simulink model "Commander_Stabilizer_Qdrone_serial"  (R2019a)
settings: Solver=ode2  StartTime=0.0  StopTime=inf  FixedStep=0.001  RelTol=1e-3  EnableMultiTasking=on
InitFcn:
  | set_param(gcs, 'ZoomFactor','FitSystem')
model workspace (MAT data in the model file):
  target_system = 1
undefined symbols (not defined in the file or in its folder): HIL, qc_get_step_size
libraries: quarc_library x53, simulink x24, simulink_extras x4
(part 2 of 4)

== system Commander_Stabilizer_Qdrone_serial/HORIZON FRAME CONVERSION AND ESTIMATION/Estimate Yaw Angle ==
  note: Improve Yaw Estimate
  note: The complementary filters for yaw estimation uses an accurate but noisy yaw approximation to correct the drifting integral of the fast gyroscopic rate to yield an accurate and fast yaw estimate.
  Yaw Rate (rad/s) : Inport
  Yaw Correction (rad) : Inport  Port=2
  Reset : Inport  Port=3
  Integrator1 : Integrator
  Integrator2 : Integrator  ExternalReset=rising
  Ki1 : Gain  Gain=0.1
  Kp1 : Gain
  Sum1 : Sum  Inputs=|-+
  Sum2 : Sum  Inputs=+--
  Yaw Estimate (rad) : Outport
  wires:
  Yaw Rate (rad/s)/1 -> Sum2/1
  Sum1/1 -> Ki1/1, Kp1/1
  Kp1/1 -> Sum2/2
  Reset/1 -> Integrator2/2
  Sum2/1 -> Integrator1/1
  Ki1/1 -> Integrator2/1
  Integrator1/1 -> Yaw Estimate (rad)/1, Sum1/2
  Integrator2/1 -> Sum2/3
  Yaw Correction (rad)/1 -> Sum1/1

== system Commander_Stabilizer_Qdrone_serial/HORIZON FRAME CONVERSION AND ESTIMATION/Pose Rate Estimation ==
  note: Second order filter + Derivative
  note: Generate Pose Rate Approximation
  note: Improve Position Rate Estimate
  note: Complementary Filter implementation (similar to those in the Stabilizer module)
  note: The complementary filter uses an accurate but noisy pose rate approximation to correct the drifting integral of the fast accelerometer readings to yield an accurate and fast pose rate estimate.
  HF Vehicle Acceleration (m/s/s) [3] : Inport
  "HF Pose Measurement (m, rad) [4]" : Inport  Port=2
  Yaw Rate (rad/s) : Inport  Port=3
  Reset : Inport  Port=4
  Integrator6 : Integrator
  Integrator7 : Integrator  ExternalReset=rising
  Ki3 : Gain  Gain=0.1
  Kp3 : Gain
  Mux2 : Mux  Inputs=2
  Second-Order Low-Pass Filter : quarc_library/Continuous/Second-Order Low-Pass Filter  params_source=External (input ports)  input_width=1  input_zeta=1  input_init=0
  Selector : Selector  InputPortWidth=4  IndexOptions=Index vector (dialog)  Indices=[1:3]  OutputSizes=1
  Sum8 : Sum  Inputs=|-+
  Sum9 : Sum  Inputs=+--
  Terminator1 : Terminator
  wn : Constant  Value=50
  zt : Constant
  "HF Pose Rate Estimate (m/s, rad/s) [4]" : Outport
  wires:
  "HF Pose Measurement (m, rad) [4]"/1 -> Selector/1
  Yaw Rate (rad/s)/1 -> Mux2/2
  Reset/1 -> Integrator7/2
  Integrator7/1 -> Sum9/3
  Integrator6/1 -> Sum8/2, Mux2/1
  Kp3/1 -> Sum9/2
  Ki3/1 -> Integrator7/1
  Sum8/1 -> Kp3/1, Ki3/1
  Sum9/1 -> Integrator6/1
  Mux2/1 -> "HF Pose Rate Estimate (m/s, rad/s) [4]"/1
  wn/1 -> Second-Order Low-Pass Filter/2
  Second-Order Low-Pass Filter/1 -> Terminator1/1
  Second-Order Low-Pass Filter/2 -> Sum8/1
  zt/1 -> Second-Order Low-Pass Filter/3
  HF Vehicle Acceleration (m/s/s) [3]/1 -> Sum9/1
  Selector/1 -> Second-Order Low-Pass Filter/4, Second-Order Low-Pass Filter/1

== system Commander_Stabilizer_Qdrone_serial/HORIZON FRAME CONVERSION AND ESTIMATION/Transform from Body Frame to Horizon Frame ==
  note: Accelerometer Reading + Gravity = Vehicle Acceleration
  HF_R_BF : Inport
  BF Net Acceleration (m/s/s) [3] : Inport  Port=2
  Product : Product  Multiplication=Matrix(*)
  gravity correction : Bias  Bias=[0 0 -9.81]
  HF Vehicle Acceleration (m/s/s) [3] : Outport
  wires:
  gravity correction/1 -> HF Vehicle Acceleration (m/s/s) [3]/1  "HF Vehicle Acceleration"
  HF_R_BF/1 -> Product/1
  BF Net Acceleration (m/s/s) [3]/1 -> Product/2
  Product/1 -> gravity correction/1  "HF Accelerometer Reading"

== system Commander_Stabilizer_Qdrone_serial/HORIZON FRAME CONVERSION AND ESTIMATION/Transform from Inertial Frame to Horizon Frame ==
  HF_R_IF : Inport
  "IF Pose Command (m, rad) [4]" : Inport  Port=2
  Yaw Estimate : Inport  Port=3
  "IF Pose Measurement (m, rad) [4]" : Inport  Port=4
  Mux1 : Mux  Inputs=2
  Mux3 : Mux  Inputs=2
  Product1 : Product  Multiplication=Matrix(*)
  Product2 : Product  Multiplication=Matrix(*)
  Select Position Command : Selector  InputPortWidth=4  IndexOptions=Index vector (dialog)  Indices=1:3  OutputSizes=1
  Select Position Estimate : Selector  InputPortWidth=4  IndexOptions=Index vector (dialog)  Indices=1:3  OutputSizes=1
  Select Yaw Command : Selector  InputPortWidth=4  IndexOptions=Index vector (dialog)  Indices=4  OutputSizes=1
  "HF Pose Estimate (m, rad) [4]" : Outport
  "HF Pose Command (m, rad) [4]" : Outport  Port=2
  wires:
  Yaw Estimate/1 -> Mux1/2
  "IF Pose Command (m, rad) [4]"/1 -> Select Position Command/1, Select Yaw Command/1
  Select Position Command/1 -> Product1/2  "IF Position Command"
  Product2/1 -> Mux1/1  "HF Position Measurement"
  Product1/1 -> Mux3/1  "HF Position Command"
  Mux3/1 -> "HF Pose Command (m, rad) [4]"/1
  Mux1/1 -> "HF Pose Estimate (m, rad) [4]"/1
  HF_R_IF/1 -> Product2/1, Product1/1
  Select Yaw Command/1 -> Mux3/2
  Select Position Estimate/1 -> Product2/2  "IF Position Measurement"
  "IF Pose Measurement (m, rad) [4]"/1 -> Select Position Estimate/1

== system Commander_Stabilizer_Qdrone_serial/STABILIZER - QDRONE /BLACKBOX ==
  Mode : Inport
  Controller Log : Inport  Port=2
  Plant Log : Inport  Port=3
  Safety Log : Inport  Port=4
  Mux : Mux
  To Host File : quarc_library/Sinks/To Host/To Host File  file_name=saved_data/%m/Stabilizer_%{date}_%{time}.mat  variable_name=stabilizer_data  decimation=1  sample_time=-1  file_format=MAT-file v.5  options=No header or footer  append=off  final_file_name=saved_data/Commander_Stabilizer_Qdrone_serial/Stabilizer_04-Apr-2021_22-18-28.mat  bitrate=2000000
      settings: SourceProductName=The database C:\Users\user\AppData\Roaming\MathWorks\MATLAB\R2017a\slblocks_master.db is locked, or a table in the database is locked. (database is locked)
  wires:
  Mux/1 -> To Host File/1
  Safety Log/1 -> Mux/1
  Controller Log/1 -> Mux/2
  Plant Log/1 -> Mux/3
  Mode/1 -> Mux/4

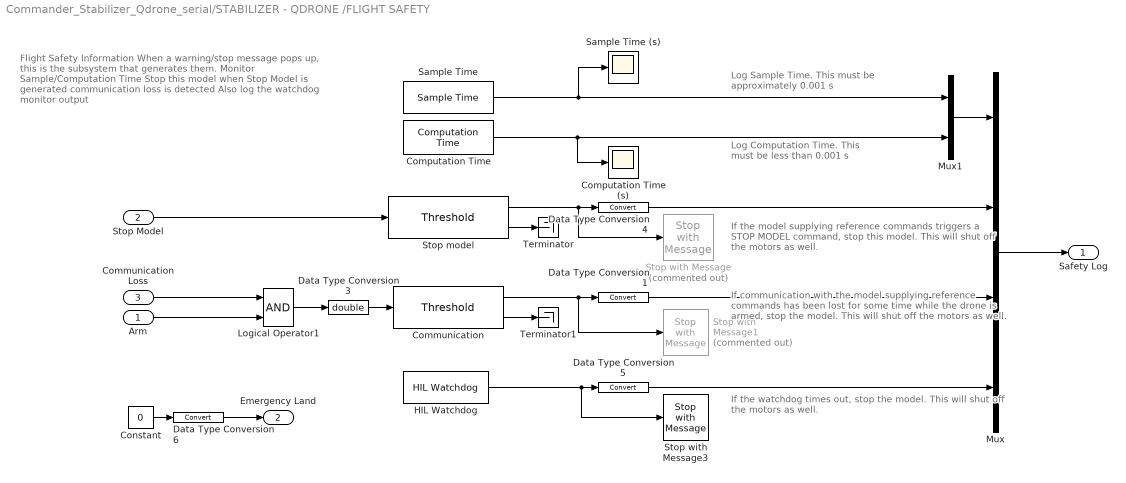
== system Commander_Stabilizer_Qdrone_serial/STABILIZER - QDRONE /FLIGHT SAFETY ==
  note: Flight Safety Information
      |
      | When a warning/stop message pops up, this is the subsystem
      | that generates them.
      |
      | Monitor Sample/Computation Time
      | Stop this model
      | when Stop Model is generated
      | communication loss is detected
      | Also log the watchdog monitor output
  note: Log Sample Time. This must be approximately 0.001 s
  note: Log Computation Time. This must be less than 0.001 s
  note: If the model supplying reference commands triggers a STOP MODEL command, stop this model. This will shut off the motors as well.
  note: If communication with the model supplying reference commands has been lost for some time while the drone is armed, stop the model. This will shut off the motors as well.
  note: If the watchdog times out, stop the model. This will shut off the motors as well.
  Arm : Inport
  Stop Model : Inport  Port=2
  Communication Loss : Inport  Port=3
  Communication : quarc_library/Discontinuities/Threshold  operator=>=  param_src=Specify via dialog  threshold=0.5  duration=1
      settings: SourceProductName=The database C:\Users\user\AppData\Roaming\MathWorks\MATLAB\R2017a\slblocks_master.db is locked, or a table in the database is locked. (database is locked)
  Computation Time : quarc_library/Sources/Time/Computation Time  sample_time=qc_get_step_size  use_model=on  use_cpu_time=off
      settings: SourceProductName=The database C:\Users\user\AppData\Roaming\MathWorks\MATLAB\R2017a\slblocks_master.db is locked, or a table in the database is locked. (database is locked)
  Computation Time (s) : Scope
  Constant : Constant  Value=0
  Data Type Conversion{1,4..6} (4 alike) : DataTypeConversion
  Data Type Conversion3 : DataTypeConversion  OutDataTypeStr=double
  HIL Watchdog : quarc_library/Data Acquisition/Generic/Watchdog/HIL Watchdog  object_name=HIL-1  timeout=0.1  sample_time=qc_get_step_size  active=off
      settings: AttributesFormatString=(%<object_name>)  SourceProductName=QUARC Targets
  Logical Operator1 : Logic  AllPortsSameDT=off  OutDataTypeStr=boolean
  Mux : Mux
  Mux1 : Mux  Inputs=2
  Sample Time : quarc_library/Sources/Time/Sample Time  Priority=-99  sample_time=qc_get_step_size
      settings: SourceProductName=The database C:\Users\user\AppData\Roaming\MathWorks\MATLAB\R2017a\slblocks_master.db is locked, or a table in the database is locked. (database is locked)
  Sample Time (s) : Scope
  Stop model : quarc_library/Discontinuities/Threshold  operator=>=  param_src=Specify via dialog  threshold=0.5  duration=0.1
      settings: SourceProductName=The database C:\Users\user\AppData\Roaming\MathWorks\MATLAB\R2017a\slblocks_master.db is locked, or a table in the database is locked. (database is locked)
  Stop with Message : quarc_library/Sinks/Error Handling/Stop with Message  Commented=on  message_type=Fixed error message  message_icon=Information  message=QDrone Stabilizer: Commander Terminated
      settings: SourceProductName=The database C:\Users\user\AppData\Roaming\MathWorks\MATLAB\R2017a\slblocks_master.db is locked, or a table in the database is locked. (database is locked)
  Stop with Message1 : quarc_library/Sinks/Error Handling/Stop with Message  Commented=on  message_type=Fixed error message  message_icon=Warning  message=QDrone Stabilizer: Communication with Commander lost
      settings: SourceProductName=The database C:\Users\user\AppData\Roaming\MathWorks\MATLAB\R2017a\slblocks_master.db is locked, or a table in the database is locked. (database is locked)
  Stop with Message3 : quarc_library/Sinks/Error Handling/Stop with Message  message_type=Fixed error message  message_icon=Information  message=QDrone Stabilizer: HIL Watchdog timer expired
      settings: SourceProductName=The database C:\Users\user\AppData\Roaming\MathWorks\MATLAB\R2017a\slblocks_master.db is locked, or a table in the database is locked. (database is locked)
  Terminator : Terminator
  Terminator1 : Terminator
  Safety Log : Outport
  Emergency Land : Outport  Port=2
  wires:
  Mux/1 -> Safety Log/1
  Computation Time/1 -> Computation Time (s)/1, Mux1/2
  Sample Time/1 -> Sample Time (s)/1, Mux1/1
  Data Type Conversion4/1 -> Mux/2
  HIL Watchdog/1 -> Stop with Message3/1, Data Type Conversion5/1
  Stop model/2 -> Terminator/1
  Stop model/1 -> Data Type Conversion4/1, Stop with Message/1
  Stop Model/1 -> Stop model/1
  Communication/2 -> Terminator1/1
  Logical Operator1/1 -> Data Type Conversion3/1
  Data Type Conversion1/1 -> Mux/3
  Arm/1 -> Logical Operator1/2
  Communication/1 -> Data Type Conversion1/1, Stop with Message1/1
  Data Type Conversion3/1 -> Communication/1
  Communication Loss/1 -> Logical Operator1/1
  Mux1/1 -> Mux/1
  Constant/1 -> Data Type Conversion6/1
  Data Type Conversion6/1 -> Emergency Land/1
  Data Type Conversion5/1 -> Mux/4

== system Commander_Stabilizer_Qdrone_serial/STABILIZER - QDRONE /MODE SWITCHBOX ==
  note: This subsystem switches between Attitude Torques AND Attitude Commands depending on
      | the value of the Mode signal:
      | Mode = 1	=> 		Torque mode, Attitude Commands are zeroed
      | Mode = 0	=> 		Angle mode, Attitude Torques are zeroed
  Mode (0,1) : Inport
  Attitude Torques : Inport  Port=2
  Attitude Commands : Inport  Port=3
  Switch : Switch  Criteria=u2 > Threshold  Threshold=0.5
  Switch1 : Switch  Criteria=u2 > Threshold  Threshold=0.5
  Zero Torque/Command : Constant  Value=[0 0 0]
  Attitude Torques (Nm) [3] : Outport
  "Attitude Commands (rad, rad/s) [3]" : Outport  Port=2
  wires:
  Zero Torque/Command/1 -> Switch1/1, Switch/3
  Attitude Torques/1 -> Switch/1
  Switch/1 -> Attitude Torques (Nm) [3]/1
  Mode (0,1)/1 -> Switch1/2, Switch/2
  Switch1/1 -> "Attitude Commands (rad, rad/s) [3]"/1
  Attitude Commands/1 -> Switch1/3

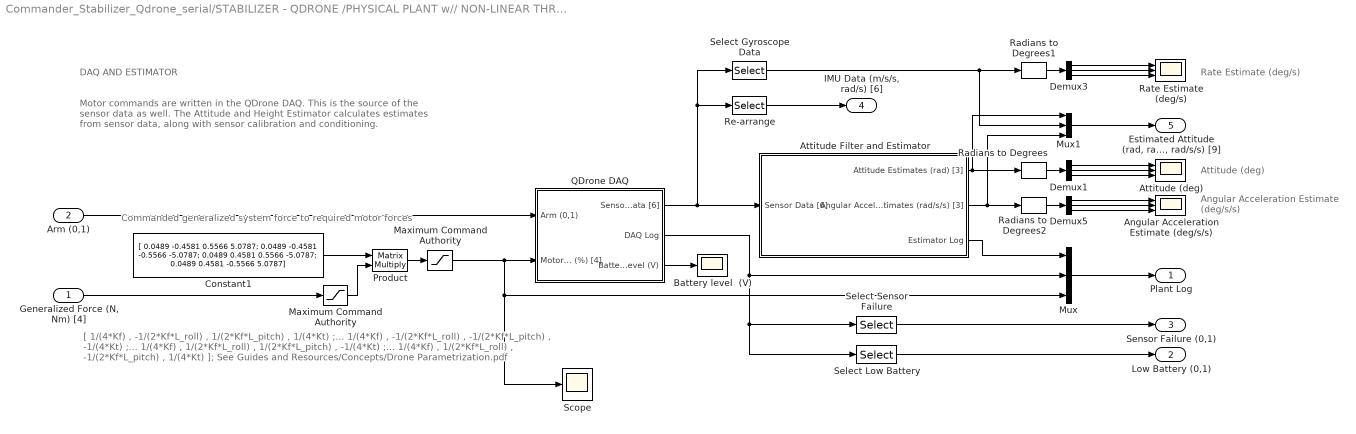
== system Commander_Stabilizer_Qdrone_serial/STABILIZER - QDRONE /PHYSICAL PLANT w// NON-LINEAR THRUST ==
  note: [ 1/(4*Kf) , -1/(2*Kf*L_roll) , 1/(2*Kf*L_pitch) , 1/(4*Kt) ;...
      | 1/(4*Kf) , -1/(2*Kf*L_roll) , -1/(2*Kf*L_pitch) , -1/(4*Kt) ;...
      | 1/(4*Kf) , 1/(2*Kf*L_roll) , 1/(2*Kf*L_pitch) , -1/(4*Kt) ;...
      | 1/(4*Kf) , 1/(2*Kf*L_roll) , -1/(2*Kf*L_pitch) , 1/(4*Kt) ];
      |
      | See Guides and Resources/Concepts/Drone Parametrization.pdf
  note: Attitude (deg)
  note: Rate Estimate (deg/s)
  note: Angular Acceleration
      | Estimate (deg/s/s)
  note: DAQ AND ESTIMATOR
  note: Motor commands are written in the QDrone DAQ. This is the source of the sensor data as well. The Attitude and Height Estimator calculates estimates from sensor data, along with sensor calibration and conditioning.
  note: Commanded generalized system force to required motor forces
  "Generalized Force (N, Nm) [4]" : Inport
  Arm (0,1) : Inport  Port=2
  Angular Acceleration Estimate (deg/s/s) : Scope  NumInputPorts=3
  Attitude (deg) : Scope  NumInputPorts=3
  Attitude Filter and Estimator : Subsystem
  Battery level  (V) : Scope
  Constant1 : Constant  Value=|
      | [ 0.0489   -0.4581    0.5566    5.0787;
      |   0.0489   -0.4581   -0.5566   -5.0787;
      |   0.0489    0.4581    0.5566   -5.0787;
      |   0.0489    0.4581   -0.5566    5.0787]
  Demux1 : Demux  Outputs=3
  Demux3 : Demux  Outputs=3
  Demux5 : Demux  Outputs=3
  Maximum Command Authority : Saturate  UpperLimit=[Inf Inf Inf Inf]  LowerLimit=[-Inf -Inf -Inf -Inf]
  "Maximum Command Authority " : Saturate  UpperLimit=[1 1 1 1]  LowerLimit=[0 0 0 0]
  Mux : Mux  Inputs=3
  Mux1 : Mux  Inputs=[3 3 3]
  Product : Product  Multiplication=Matrix(*)
  QDrone DAQ : Subsystem
  Radians to Degrees : simulink_extras/Transformations/Radians to Degrees
  Radians to Degrees1 : simulink_extras/Transformations/Radians to Degrees
  Radians to Degrees2 : simulink_extras/Transformations/Radians to Degrees
  Rate Estimate (deg/s) : Scope  NumInputPorts=3
  Re-arrange : Selector  InputPortWidth=6  IndexOptions=Index vector (dialog)  Indices=[4:6 1:3]  OutputSizes=1
  Scope : Scope
  Select Gyroscope Data : Selector  InputPortWidth=6  IndexOptions=Index vector (dialog)  Indices=[1:3]  OutputSizes=1
  Select Low Battery : Selector  InputPortWidth=9  IndexOptions=Index vector (dialog)  Indices=[3]  OutputSizes=1
  Select Sensor Failure : Selector  InputPortWidth=9  IndexOptions=Index vector (dialog)  Indices=[1]  OutputSizes=1
  Plant Log : Outport
  Low Battery (0,1) : Outport  Port=2
  Sensor Failure (0,1) : Outport  Port=3
  "IMU Data (m/s/s, rad/s) [6]" : Outport  Port=4
  "Estimated Attitude (rad, rad/s, rad/s/s) [9]" : Outport  Port=5
  wires:
  Mux/1 -> Plant Log/1
  Demux1/1 -> Attitude (deg)/1
  Demux1/2 -> Attitude (deg)/2
  Demux1/3 -> Attitude (deg)/3
  Demux3/1 -> Rate Estimate (deg/s)/1
  Demux3/2 -> Rate Estimate (deg/s)/2
  Demux3/3 -> Rate Estimate (deg/s)/3
  Demux5/1 -> Angular Acceleration Estimate (deg/s/s)/1
  Demux5/2 -> Angular Acceleration Estimate (deg/s/s)/2
  Demux5/3 -> Angular Acceleration Estimate (deg/s/s)/3
  Attitude Filter and Estimator/3(Estimator Log) -> Mux/1
  Arm (0,1)/1 -> QDrone DAQ/1(Arm (0,1))
  QDrone DAQ/2(DAQ Log) -> Select Sensor Failure/1, Select Low Battery/1, Mux/2
  Select Low Battery/1 -> Low Battery (0,1)/1
  Select Sensor Failure/1 -> Sensor Failure (0,1)/1
  Radians to Degrees/1 -> Demux1/1
  Radians to Degrees1/1 -> Demux3/1
  Radians to Degrees2/1 -> Demux5/1
  "Maximum Command Authority "/1 -> Scope/1, Mux/3, QDrone DAQ/2(Motor Cmd (%) [4])
  Attitude Filter and Estimator/1(Attitude Estimates (rad) [3]) -> Mux1/1, Radians to Degrees/1
  Select Gyroscope Data/1 -> Radians to Degrees1/1, Mux1/2
  Mux1/1 -> "Estimated Attitude (rad, rad/s, rad/s/s) [9]"/1
  QDrone DAQ/3(Battery Level (V)) -> Battery level  (V)/1
  Attitude Filter and Estimator/2(Angular Accel. Estimates (rad/s/s) [3]) -> Mux1/3, Radians to Degrees2/1
  Constant1/1 -> Product/1
  Maximum Command Authority/1 -> Product/2
  "Generalized Force (N, Nm) [4]"/1 -> Maximum Command Authority/1
  Product/1 -> "Maximum Command Authority "/1
  Re-arrange/1 -> "IMU Data (m/s/s, rad/s) [6]"/1
  QDrone DAQ/1(Sensor Data [6]) -> Re-arrange/1, Select Gyroscope Data/1, Attitude Filter and Estimator/1(Sensor Data [6])

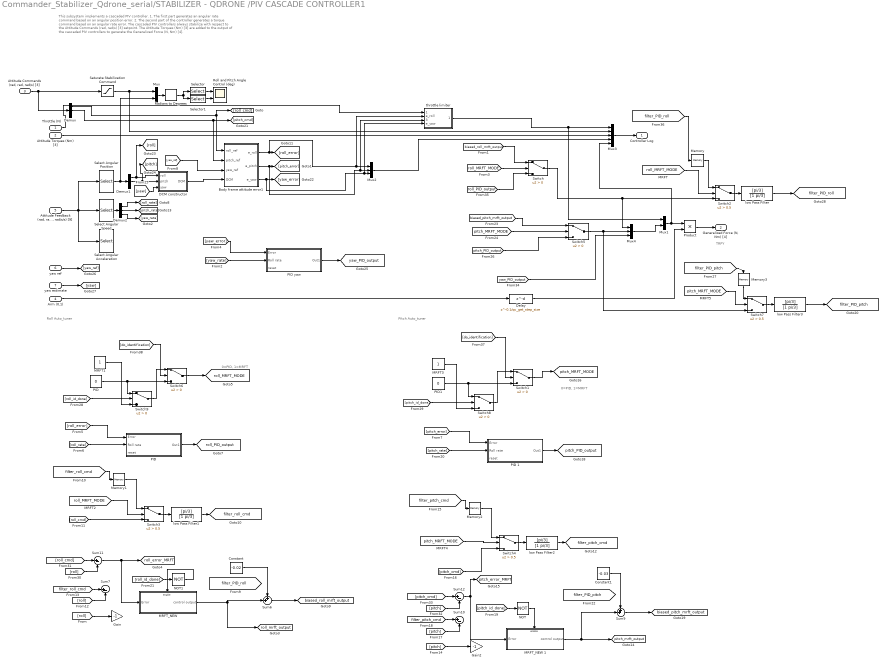
== system Commander_Stabilizer_Qdrone_serial/STABILIZER - QDRONE /PIV CASCADE CONTROLLER1 ==
  note: This subsystem implements a cascaded PIV controller.
      | 1. The first part generates an angular rate command based on an angular position error.
      | 2. The second part of the controller generates a torque command based on an angular rate error.
      |
      | The cascaded PIV controllers always stabilize with respect to the Attitude Commands (rad, rad/s) [3] setpoint. The Attitude Torques (Nm) [3] are added to the output of the cascaded PIV controllers to generate the Generalized Force (N, Nm) [4].
  note: 0=PID, 1=MRFT
  note: Roll Auto_tuner
  note: Pitch Auto_tuner
  note: TRPY
  note: 0=PID, 1=MRFT
  Throttle (N) : Inport
  Attitude Torques (Nm) [3] : Inport  Port=2
  "Attitude Commands (rad, rad, rad/s) [3]" : Inport  Port=3
  Arm (0,1) : Inport  Port=4
  "Attitude Feedback (rad, rad/s, rad/s/s) [9]" : Inport  Port=5
  "yaw ref " : Inport  Port=6
  "yaw estimate " : Inport  Port=7
  Body frame attitude error1 : MATLAB Function  TreatAsAtomicUnit=on
  Constant : Constant  Value=-0.02
  Constant1 : Constant  Value=-0.03
  "DCM constructor " : MATLAB Function  TreatAsAtomicUnit=on
  Delay : Delay  DelayLength=0.1/qc_get_step_size
  Demux : Demux  Outputs=3
  Demux1 : Demux  Outputs=3
  Demux2 : Demux  Outputs=3
  Gain : Gain  Gain=-1
  Gain2 : Gain  Gain=-1
  MRFT1 : Constant
  MRFT3 : Constant
  "MRFT_NEW " : Subsystem
  MRFT_NEW 1 : Subsystem
  Memory{,1..3} (4 alike) : Memory
  Mux : Mux  Inputs=2
  Mux1 : Mux  Inputs=2
  Mux2 : Mux  Inputs=3
  Mux3 : Mux  Inputs=5
  Mux4 : Mux  Inputs=3
  NOT : Logic  Operator=NOT  IconShape=distinctive  AllPortsSameDT=off  OutDataTypeStr=boolean
  NOT1 : Logic  Operator=NOT  IconShape=distinctive  AllPortsSameDT=off  OutDataTypeStr=boolean
  PID : Constant  Value=0
  "PID " : Subsystem
  PID 1 : Subsystem
  PID yaw : Subsystem
  PID1 : Constant  Value=0
  Product : Product
  Radians to Degrees : simulink_extras/Transformations/Radians to Degrees
  Roll and Pitch Angle Control (deg) : Scope  NumInputPorts=2
  Saturate Stabilization Command : Saturate  UpperLimit=[pi/2 pi/2 10*pi/18]  LowerLimit=[-pi/2 -pi/2 -10*pi/18]
  Select Angular Acceleration : Selector  InputPortWidth=9  IndexOptions=Index vector (dialog)  Indices=[7:9]  OutputSizes=1
  Select Angular Speed : Selector  InputPortWidth=9  IndexOptions=Index vector (dialog)  Indices=[4:6]  OutputSizes=1
  Select Angular Position : Selector  InputPortWidth=9  IndexOptions=Index vector (dialog)  Indices=[1:3]  OutputSizes=1
  Selector : Selector  InputPortWidth=6  IndexOptions=Index vector (dialog)  Indices=[1 4]  OutputSizes=1
  Selector1 : Selector  InputPortWidth=6  IndexOptions=Index vector (dialog)  Indices=[2 5]  OutputSizes=1
  Sum{7,10..12} (4 alike) : Sum  Inputs=|+-
  Sum6 : Sum  Inputs=++|
  Sum9 : Sum  Inputs=++|
  Switch{,1,5..6,8..9} (6 alike) : Switch  Criteria=u2 > Threshold
  Switch{2..4,7} (4 alike) : Switch  Criteria=u2 > Threshold  Threshold=0.5
  low Pass Filter{,1..3} (4 alike) : TransferFcn  Numerator=[pi/3]  Denominator=[1 pi/3]
  throttle limiter : MATLAB Function  TreatAsAtomicUnit=on
  Controller Log : Outport
  "Generalized Force (N, Nm) [4]" : Outport  Port=2
  tag scope: biased_pitch_mrft_output=global, biased_roll_mrft_output=global, filter_PID_pitch=global, filter_PID_roll=global, filter_pitch_cmd=global, filter_roll_cmd=global, pitch_MRFT_MODE=global, pitch_PID_output=global, pitch_error_MRFT=global, pitch_mrft_output=global, roll_MRFT_MODE=global, roll_PID_output=global, roll_error_MRFT=global, roll_mrft_output=global, yaw_PID_output=global
  wires:
  [roll] -> Gain/1
  "MRFT_NEW "/1(control output) -> Sum6/2, [roll_mrft_output]
  PID/1 -> Switch9/1, Switch6/3
  MRFT1/1 -> Switch9/3
  Sum6/1 -> [biased_roll_mrft_output]
  low Pass Filter1/1 -> [filter_roll_cmd]
  [roll_MRFT_MODE] -> Switch3/2
  Memory1/1 -> Switch3/1
  Switch3/1 -> low Pass Filter1/1
  [roll_cmd] -> Switch3/3
  [filter_roll_cmd] -> Memory1/1
  [filter_roll_cmd] -> Sum7/1
  [roll] -> Sum7/2
  [pitch_cmd] -> Switch4/3
  [pitch] -> Sum10/2
  [filter_pitch_cmd] -> Sum10/1
  Switch4/1 -> low Pass Filter2/1
  Memory2/1 -> Switch4/1
  Sum9/1 -> [biased_pitch_mrft_output]
  [filter_pitch_cmd] -> Memory2/1
  low Pass Filter2/1 -> [filter_pitch_cmd]
  [pitch_MRFT_MODE] -> Switch4/2
  MRFT_NEW 1/1(control output) -> Sum9/2, [pitch_mrft_output]
  [pitch] -> Gain2/1
  [roll_id_done] -> Switch9/2
  Switch9/1 -> Switch6/1
  [roll] -> Sum11/2
  [roll_cmd] -> Sum11/1
  [pitch_cmd] -> Sum12/1
  [pitch] -> Sum12/2
  Sum11/1 -> "MRFT_NEW "/1(Error), [roll_error_MRFT]
  Sum12/1 -> MRFT_NEW 1/1(Error), [pitch_error_MRFT]
  PID yaw/1(Out1) -> [yaw_PID_output]
  Demux/2 -> [pitch_cmd], Body frame attitude error1/2(pitch_ref)
  [yaw_rate] -> PID yaw/2(Roll rate)
  "yaw ref "/1 -> [yaw_ref]
  "yaw estimate "/1 -> [yaw]
  Demux1/2 -> [pitch], "DCM constructor "/2(pitch)
  Throttle (N)/1 -> throttle limiter/1(throttle_in)
  [yaw_error] -> PID yaw/1(Error)
  Demux/1 -> Body frame attitude error1/1(roll_ref), [roll_cmd]
  throttle limiter/1(throttle_out) -> Mux1/1, Mux3/1
  "Attitude Feedback (rad, rad/s, rad/s/s) [9]"/1 -> Select Angular Speed/1, Select Angular Position/1, Select Angular Acceleration/1
  Arm (0,1)/1 -> Delay/1
  Product/1 -> "Generalized Force (N, Nm) [4]"/1
  [pitch_MRFT_MODE] -> Switch7/2
  Body frame attitude error1/3(e_yaw) -> throttle limiter/4(e_yaw), Mux2/3, [yaw_error]
  Mux2/1 -> Mux3/4
  Demux1/1 -> [roll], "DCM constructor "/1(roll)
  Mux4/1 -> Mux1/2
  "DCM constructor "/1(DCM) -> Body frame attitude error1/4(DCM)
  Switch5/1 -> Switch7/3, Mux4/2
  Attitude Torques (Nm) [3]/1 -> Mux3/3
  Select Angular Speed/1 -> Demux2/1
  [pitch_MRFT_MODE] -> Switch5/2
  "Attitude Commands (rad, rad, rad/s) [3]"/1 -> Saturate Stabilization Command/1, Demux/1
  [yaw_ref] -> Body frame attitude error1/3(yaw_ref)
  [filter_PID_pitch] -> Memory3/1
  Switch7/1 -> low Pass Filter3/1
  Selector1/1 -> Roll and Pitch Angle Control (deg)/2
  Demux2/2 -> [pitch_rate]
  Memory3/1 -> Switch7/1
  [pitch_PID_output] -> Switch5/3
  Mux/1 -> Radians to Degrees/1
  Body frame attitude error1/1(e_roll) -> throttle limiter/2(e_roll), Mux2/1, [roll_error]
  Saturate Stabilization Command/1 -> Mux/1, Mux3/2
  Radians to Degrees/1 -> Selector/1, Selector1/1
  Selector/1 -> Roll and Pitch Angle Control (deg)/1
  Switch/1 -> Mux4/1, Switch2/3
  Demux2/3 -> [yaw_rate]
  [filter_PID_roll] -> Memory/1
  Demux2/1 -> [roll_rate]
  [yaw_PID_output] -> Mux4/3
  low Pass Filter/1 -> [filter_PID_roll]
  [roll_MRFT_MODE] -> Switch2/2
  [biased_pitch_mrft_output] -> Switch5/1
  [roll_PID_output] -> Switch/3
  [biased_roll_mrft_output] -> Switch/1
  [yaw] -> "DCM constructor "/3(yaw)
  Mux3/1 -> Controller Log/1
  Memory/1 -> Switch2/1
  Delay/1 -> Product/2
  Mux1/1 -> Mux3/5, Product/1
  Switch2/1 -> low Pass Filter/1
  Select Angular Position/1 -> Demux1/1, Mux/2
  [roll_MRFT_MODE] -> Switch/2
  Body frame attitude error1/2(e_pitch) -> throttle limiter/3(e_pitch), Mux2/2, [pitch_error]
  low Pass Filter3/1 -> [filter_PID_pitch]
  [do_identification] -> Switch1/2
  Switch1/1 -> [pitch_MRFT_MODE]
  [pitch_id_done] -> Switch8/2
  Switch8/1 -> Switch1/1
  PID1/1 -> Switch8/1, Switch1/3
  MRFT3/1 -> Switch8/3
  [do_identification] -> Switch6/2
  Switch6/1 -> [roll_MRFT_MODE]
  Constant/1 -> Sum6/1
  Constant1/1 -> Sum9/1
  [roll_error] -> "PID "/1(Error)
  "PID "/1(Out1) -> [roll_PID_output]
  [roll_rate] -> "PID "/2(Roll rate)
  PID 1/1(Out1) -> [pitch_PID_output]
  [pitch_error] -> PID 1/1(Error)
  [pitch_rate] -> PID 1/2(Roll rate)
  [pitch_id_done] -> NOT/1
  NOT/1 -> MRFT_NEW 1/Enable
  NOT1/1 -> "MRFT_NEW "/Enable
  [roll_id_done] -> NOT1/1

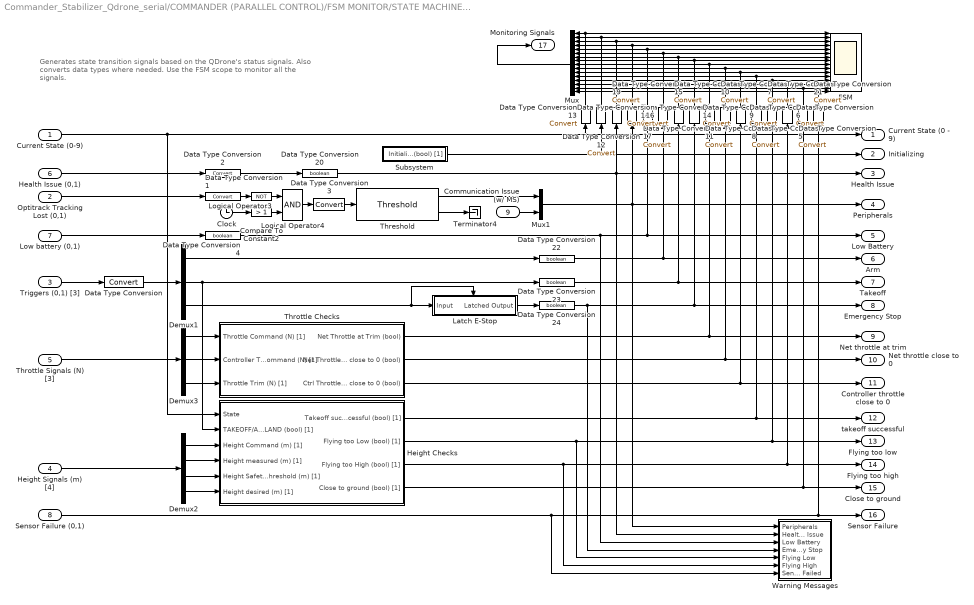
== system Commander_Stabilizer_Qdrone_serial/COMMANDER (PARALLEL CONTROL)/FSM MONITOR/STATE MACHINE SIGNALS ==
  note: Generates state transition signals based on the QDrone's status signals.
      | Also converts data types where needed.
      |
      | Use the FSM scope to monitor all the signals.
  Current State (0-9) : Inport
  "Optitrack Tracking Lost (0,1)  " : Inport  Port=2
  Triggers (0,1) [3] : Inport  Port=3
  Height Signals (m) [4] : Inport  Port=4
  Throttle Signals (N) [3] : Inport  Port=5
  "Health Issue (0,1)  " : Inport  Port=6
  Low battery (0,1) : Inport  Port=7
  Sensor Failure (0,1) : Inport  Port=8
  Communication Issue (w/ MS) : Inport  Port=9
  Clock : Clock
  Compare To Constant2 : simulink/Logic and Bit Operations/Compare To Constant  relop=>  const=1  OutDataTypeStr=boolean
  Data Type Conversion{,1..3,5..19,21} (20 alike) : DataTypeConversion
  Data Type Conversion{4,20,22..24} (5 alike) : DataTypeConversion  OutDataTypeStr=boolean
  Demux1 : Demux  Outputs=3
  Demux2 : Demux
  Demux3 : Demux  Outputs=3
  FSM : Scope  NumInputPorts=16
  Height Checks : Subsystem
  Latch E-Stop : Subsystem  TreatAsAtomicUnit=on
  Logical Operator3 : Logic  Operator=NOT  AllPortsSameDT=off  OutDataTypeStr=boolean
  Logical Operator4 : Logic  AllPortsSameDT=off  OutDataTypeStr=boolean
  Mux : Mux  Inputs=16
  Mux1 : Mux  Inputs=2
  Subsystem : Subsystem
  Terminator4 : Terminator
  Threshold : quarc_library/Discontinuities/Threshold  operator=>=  param_src=Specify via dialog  threshold=0.5  duration=0.2
      settings: SourceProductName=QUARC Targets
  Throttle Checks : Subsystem
  Warning Messages : Subsystem
  "Current State (0 - 9)  " : Outport
  Initializing : Outport  Port=2
  Health Issue : Outport  Port=3
  Peripherals : Outport  Port=4
  Low Battery : Outport  Port=5
  Arm : Outport  Port=6
  Takeoff : Outport  Port=7
  Emergency Stop : Outport  Port=8
  Net throttle at trim : Outport  Port=9
  Net throttle close to 0 : Outport  Port=10
  Controller throttle close to 0 : Outport  Port=11
  takeoff successful : Outport  Port=12
  Flying too low : Outport  Port=13
  Flying too high : Outport  Port=14
  Close to ground : Outport  Port=15
  "  Sensor Failure" : Outport  Port=16
  Monitoring Signals : Outport  Port=17
  wires:
  Triggers (0,1) [3]/1 -> Data Type Conversion/1
  Demux2/1 -> Height Checks/3(Height Command (m) [1])
  Demux3/1 -> Throttle Checks/1(Throttle Command (N) [1])
  Height Signals (m) [4]/1 -> Demux2/1
  Demux2/4 -> Height Checks/6(Height desired (m) [1])
  Throttle Signals (N) [3]/1 -> Demux3/1
  Throttle Checks/3(Ctrl Throttle close to 0 (bool)) -> Data Type Conversion9/1, Controller throttle close to 0/1
  Demux1/1 -> Data Type Conversion22/1
  Throttle Checks/2(Net Throttle close to 0 (bool)) -> Data Type Conversion10/1, Net throttle close to 0/1
  Height Checks/1(Takeoff successful (bool) [1]) -> Data Type Conversion8/1, takeoff successful/1
  Demux2/3 -> Height Checks/5(Height Safety Threshold (m) [1])
  Demux1/2 -> Height Checks/2(TAKEOFF/AUTOLAND (bool) [1]), Data Type Conversion23/1
  Demux2/2 -> Height Checks/4(Height measured (m) [1])
  Demux3/2 -> Throttle Checks/2(Controller Throttle Command (N) [1])
  Demux3/3 -> Throttle Checks/3(Throttle Trim (N) [1])
  Throttle Checks/1(Net Throttle at Trim (bool)) -> Data Type Conversion11/1, Net throttle at trim/1
  Height Checks/3(Flying too High (bool) [1]) -> Warning Messages/6(Flying High), Data Type Conversion6/1, Flying too high/1
  Height Checks/4(Close to ground (bool) [1]) -> Data Type Conversion5/1, Close to ground/1
  Data Type Conversion/1 -> Demux1/1
  "Health Issue (0,1)  "/1 -> Data Type Conversion2/1
  Low battery (0,1)/1 -> Data Type Conversion4/1
  Height Checks/2(Flying too Low (bool) [1]) -> Warning Messages/5(Flying Low), Data Type Conversion7/1, Flying too low/1
  Sensor Failure (0,1)/1 -> Data Type Conversion21/1, "  Sensor Failure"/1, Warning Messages/7(Sensor Failed)
  Mux1/1 -> Data Type Conversion18/1, Warning Messages/1(Peripherals), Peripherals/1
  Subsystem/1(Initializing (bool) [1]) -> Data Type Conversion12/1, Initializing/1
  Communication Issue (w/ MS)/1 -> Mux1/2
  Data Type Conversion1/1 -> Logical Operator3/1
  Data Type Conversion3/1 -> Threshold/1
  Compare To Constant2/1 -> Logical Operator4/2
  Clock/1 -> Compare To Constant2/1
  Logical Operator4/1 -> Data Type Conversion3/1
  Threshold/2 -> Terminator4/1
  Logical Operator3/1 -> Logical Operator4/1
  Threshold/1 -> Mux1/1
  "Optitrack Tracking Lost (0,1)  "/1 -> Data Type Conversion1/1
  Current State (0-9)/1 -> Data Type Conversion13/1, "Current State (0 - 9)  "/1, Height Checks/1(State)
  Data Type Conversion2/1 -> Data Type Conversion20/1
  Data Type Conversion4/1 -> Warning Messages/3(Low Battery), Data Type Conversion17/1, Low Battery/1
  Mux/1 -> Monitoring Signals/1
  Data Type Conversion13/1 -> Mux/1, FSM/1
  Data Type Conversion12/1 -> Mux/2, FSM/2
  Data Type Conversion19/1 -> Mux/3, FSM/3
  Data Type Conversion18/1 -> Mux/4, FSM/4
  Data Type Conversion17/1 -> Mux/5, FSM/5
  Data Type Conversion16/1 -> Mux/6, FSM/6
  Data Type Conversion15/1 -> Mux/7, FSM/7
  Data Type Conversion14/1 -> Mux/8, FSM/8
  Data Type Conversion11/1 -> Mux/9, FSM/9
  Data Type Conversion10/1 -> Mux/10, FSM/10
  Data Type Conversion9/1 -> Mux/11, FSM/11
  Data Type Conversion8/1 -> Mux/12, FSM/12
  Data Type Conversion7/1 -> Mux/13, FSM/13
  Data Type Conversion6/1 -> Mux/14, FSM/14
  Data Type Conversion5/1 -> FSM/15, Mux/15
  Data Type Conversion21/1 -> FSM/16, Mux/16
  Data Type Conversion20/1 -> Data Type Conversion19/1, Warning Messages/2(Health Issue), Health Issue/1
  Data Type Conversion22/1 -> Data Type Conversion16/1, Arm/1
  Data Type Conversion23/1 -> Data Type Conversion15/1, Takeoff/1
  Data Type Conversion24/1 -> Warning Messages/4("Emergency Stop "), Data Type Conversion14/1, Emergency Stop/1
  Latch E-Stop/1(Latched Output) -> Data Type Conversion24/1
  Demux1/3 -> Latch E-Stop/Trigger, Latch E-Stop/1(Input)

== system Commander_Stabilizer_Qdrone_serial/COMMANDER (PARALLEL CONTROL)/POSE SWITCHBOX/Use des height when enabled ==
  h_d (m) [1] : Inport
  Enable : EnablePort
  Out1 : Outport  OutputWhenDisabled=reset  InitialOutput=0
  wires:
  h_d (m) [1]/1 -> Out1/1

== system Commander_Stabilizer_Qdrone_serial/COMMANDER (PARALLEL CONTROL)/POSE SWITCHBOX/Use des yaw when enabled ==
  h_d (m) [1] : Inport
  Enable : EnablePort
  Out1 : Outport  OutputWhenDisabled=reset  InitialOutput=0
  wires:
  h_d (m) [1]/1 -> Out1/1

== system Commander_Stabilizer_Qdrone_serial/COMMANDER (PARALLEL CONTROL)/POSE SWITCHBOX/Use desired X when enabled ==
  h_d (m) [1] : Inport
  Enable : EnablePort
  Out1 : Outport  OutputWhenDisabled=reset  InitialOutput=0
  wires:
  h_d (m) [1]/1 -> Out1/1

== system Commander_Stabilizer_Qdrone_serial/COMMANDER (PARALLEL CONTROL)/POSE SWITCHBOX/Use desired Y when enabled ==
  h_d (m) [1] : Inport
  Enable : EnablePort
  Out1 : Outport  OutputWhenDisabled=reset  InitialOutput=0
  wires:
  h_d (m) [1]/1 -> Out1/1

== system Commander_Stabilizer_Qdrone_serial/COMMANDER (PARALLEL CONTROL)/THROTTLE SWITCHBOX /Use desired height when enabled ==
  h_d (m) [1] : Inport
  Enable : EnablePort
  Out1 : Outport  OutputWhenDisabled=reset  InitialOutput=0
  wires:
  h_d (m) [1]/1 -> Out1/1

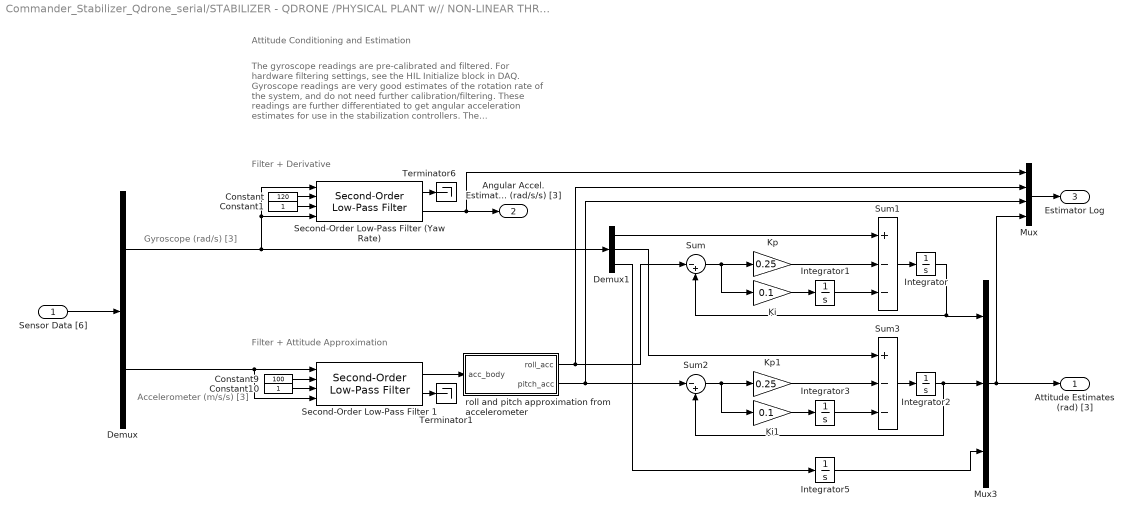
== system Commander_Stabilizer_Qdrone_serial/STABILIZER - QDRONE /PHYSICAL PLANT w// NON-LINEAR THRUST/Attitude Filter and Estimator ==
  note: Filter + Derivative
  note: Attitude Conditioning and Estimation
  note: Gyroscope (rad/s) [3]
  note: Accelerometer (m/s/s) [3]
  note: The gyroscope readings are pre-calibrated and filtered. For hardware filtering settings, see the HIL Initialize block in DAQ. Gyroscope readings are very good estimates of the rotation rate of the system, and do not need further calibration/filtering. These readings are further differentiated to get angular acceleration estimates for use in the stabilization controllers.
      |
      | The accelerometer readings in body reference frame are used to calculate a roll and pitch approximation. This is based on the knowledge that the gravity vector points straight down.
  note: Filter + Attitude Approximation
  Sensor Data [6] : Inport
  Constant : Constant  Value=120
  Constant1 : Constant
  Constant10 : Constant
  Constant9 : Constant  Value=100
  Demux : Demux  Outputs=[3 3]
  Demux1 : Demux  Outputs=3
  Integrator{,1..3,5} (5 alike) : Integrator
  Ki : Gain  Gain=0.1
  Ki1 : Gain  Gain=0.1
  Kp : Gain  Gain=0.25
  Kp1 : Gain  Gain=0.25
  Mux : Mux
  Mux3 : Mux  Inputs=3
  Second-Order Low-Pass Filter (Yaw Rate) : quarc_library/Continuous/Second-Order Low-Pass Filter  params_source=External (input ports)  input_width=200  input_zeta=1  input_init=0
      settings: SourceProductName=The database C:\Users\user\AppData\Roaming\MathWorks\MATLAB\R2017a\slblocks_master.db is locked, or a table in the database is locked. (database is locked)
  Second-Order Low-Pass Filter 1 : quarc_library/Continuous/Second-Order Low-Pass Filter  params_source=External (input ports)  input_width=50  input_zeta=1  input_init=0
      settings: SourceProductName=The database C:\Users\user\AppData\Roaming\MathWorks\MATLAB\R2017a\slblocks_master.db is locked, or a table in the database is locked. (database is locked)
  Sum : Sum  Inputs=|-+
  Sum1 : Sum  Inputs=+--
  Sum2 : Sum  Inputs=|-+
  Sum3 : Sum  Inputs=+--
  Terminator1 : Terminator
  Terminator6 : Terminator
  roll and pitch approximation from accelerometer : MATLAB Function  TreatAsAtomicUnit=on
  Attitude Estimates (rad) [3] : Outport
  Angular Accel. Estimates (rad/s/s) [3] : Outport  Port=2
  Estimator Log : Outport  Port=3
  wires:
  Sensor Data [6]/1 -> Demux/1
  Mux3/1 -> Mux/4, Attitude Estimates (rad) [3]/1
  Second-Order Low-Pass Filter (Yaw Rate)/2 -> Mux/1, Angular Accel. Estimates (rad/s/s) [3]/1
  Mux/1 -> Estimator Log/1
  Second-Order Low-Pass Filter 1/2 -> Terminator1/1
  Constant9/1 -> Second-Order Low-Pass Filter 1/2
  Constant10/1 -> Second-Order Low-Pass Filter 1/3
  Second-Order Low-Pass Filter (Yaw Rate)/1 -> Terminator6/1
  Demux/2 -> Second-Order Low-Pass Filter 1/4, Second-Order Low-Pass Filter 1/1
  roll and pitch approximation from accelerometer/2(pitch_acc) -> Mux/3, Sum2/1
  roll and pitch approximation from accelerometer/1(roll_acc) -> Sum/1, Mux/2
  Constant/1 -> Second-Order Low-Pass Filter (Yaw Rate)/2
  Second-Order Low-Pass Filter 1/1 -> roll and pitch approximation from accelerometer/1(acc_body)
  Constant1/1 -> Second-Order Low-Pass Filter (Yaw Rate)/3
  Demux1/3 -> Integrator5/1
  Integrator1/1 -> Sum1/3
  Integrator/1 -> Sum/2, Mux3/1
  Sum1/1 -> Integrator/1
  Kp/1 -> Sum1/2
  Sum/1 -> Ki/1, Kp/1
  Ki/1 -> Integrator1/1
  Demux1/1 -> Sum1/1
  Demux/1 -> Second-Order Low-Pass Filter (Yaw Rate)/1, Second-Order Low-Pass Filter (Yaw Rate)/4, Demux1/1
  Integrator5/1 -> Mux3/3
  Ki1/1 -> Integrator3/1
  Sum2/1 -> Kp1/1, Ki1/1
  Kp1/1 -> Sum3/2
  Sum3/1 -> Integrator2/1
  Integrator2/1 -> Sum2/2, Mux3/2
  Integrator3/1 -> Sum3/3
  Demux1/2 -> Sum3/1

== system Commander_Stabilizer_Qdrone_serial/STABILIZER - QDRONE /PHYSICAL PLANT w// NON-LINEAR THRUST/QDrone DAQ ==
  note: Read the sensors and battery voltage
  note: Write to motors and LEDs
  note: DAQ
  note: Motor commands are written to the QDrone via the HIL Write block. The motor command inputs are mapped for a Oneshot 125 protocol as follows:
      |
      | Percent Seconds Description
      | 0% 125 us No Throttle
      | 100% 250 us Max Throttle
      |
      | The input to the motors are written as time period (in seconds) of the PWM pulses (at 2kHz).
      |
      | LED colors can be set using a simple 3x1 ON (1) and OFF (0) vector (RGB mode).
  note: Gyro and Accel data rate at 1000Hz
  Arm (0,1) : Inport
  Motor Cmd (%) [4] : Inport  Port=2
  Accel (m/s/s) [3] : Selector  InputPortWidth=6  IndexOptions=Index vector (dialog)  Indices=[4:6]  OutputSizes=1
  "Battery Level, Accelrometer and Gyroscope" : quarc_library/Data Acquisition/Generic/Immediate I//O/HIL Read  Priority=1  object_name=HIL-1  analog_channels=[4]  encoder_channels=[]  digital_channels=[]  other_channels=[3000:3002 4000:4002]  sample_time=qc_get_step_size  active=on  vector_output=on  data_type_mode=Inherit via back propagation  encoder_data_type=double  digital_data_type=boolean
      settings: SourceProductName=The database C:\Users\user\AppData\Roaming\MathWorks\MATLAB\R2017a\slblocks_master.db is locked, or a table in the database is locked. (database is locked)
  Bias - Pulse Offset (%) : Bias  Bias=125e-6
  Check Battery level : Subsystem
  Conversion : Gain  Gain=11.2
  Gyro (rad/s) [3] : Selector  InputPortWidth=6  IndexOptions=Index vector (dialog)  Indices=[1:3]  OutputSizes=1
  HIL Initialize : quarc_library/Data Acquisition/Generic/Configuration/HIL Initialize  object_name=HIL-1  board_type=qdrone  board_number=0  board_options=gyro_fs=2000;gyro_rate=1000;gyro_os=4;accel_fs=16;accel_rate=400;accel_os=4;baro_os=4096  exclusive=off  active=on  hardware_clocks=[]  clock_modes=[]  initial_clock_frequencies=[]  set_clock_params_at_start=off  set_clock_params_at_switch_in=off  set_clock_frequencies_at_start=off  set_clock_frequencies_at_switch_in=off  analog_input_channels=[0:4]  analog_input_configurations=[]  analog_input_maximums=[3.3]  analog_input_minimums=[0]  set_analog_input_params_at_start=off  set_analog_input_params_at_switch_in=off  analog_output_channels=[]  analog_output_maximums=[]  analog_output_minimums=[]  initial_analog_outputs=[]  final_analog_outputs=[]  watchdog_analog_outputs=[]  set_analog_output_params_at_start=off  set_analog_output_params_at_switch_in=off  set_analog_outputs_at_start=off  set_analog_outputs_at_switch_in=off  set_analog_outputs_at_terminate=off  set_analog_outputs_at_switch_out=off  set_analog_outputs_on_watchdog=off  digital_input_channels=[]  digital_output_channels=[5:7 9:23]  digital_output_configuration=[]  initial_digital_outputs=[0]  final_digital_outputs=[0]  watchdog_digital_outputs=[]  set_digital_output_params_at_start=off  set_digital_output_params_at_switch_in=off  set_digital_outputs_at_start=on  set_digital_outputs_at_switch_in=off  set_digital_outputs_at_terminate=on  set_digital_outputs_at_switch_out=off  set_digital_outputs_on_watchdog=off  encoder_channels=[0:2]  quadrature=[4]  encoder_filter_frequency=50e6/1  initial_encoder_counts=[0]  set_encoder_params_at_start=on  set_encoder_params_at_switch_in=off  set_encoder_counts_at_start=on  set_encoder_counts_at_switch_in=off  pwm_channels=[0:3]  pwm_modes=[4]  pwm_frequency=2000  pwm_configuration=[0]  pwm_alignment=[0]  pwm_polarity=[1]  pwm_leading_deadband=[]  pwm_trailing_deadband=[]  initial_pwm_outputs=[0]  final_pwm_outputs=[0]  watchdog_pwm_outputs=[0]  set_pwm_params_at_start=on  set_pwm_params_at_switch_in=off  set_pwm_outputs_at_start=on  set_pwm_outputs_at_switch_in=off  set_pwm_outputs_at_terminate=on  set_pwm_outputs_at_switch_out=off  set_pwm_outputs_on_watchdog=off  other_output_channels=[]  initial_other_outputs=[]  final_other_outputs=[]  watchdog_other_outputs=[]  set_other_outputs_at_start=off  set_other_outputs_at_switch_in=off  set_other_outputs_at_terminate=off  set_other_outputs_at_switch_out=off  set_other_outputs_on_watchdog=off
      settings: SourceProductName=The database C:\Users\user\AppData\Roaming\MathWorks\MATLAB\R2017a\slblocks_master.db is locked, or a table in the database is locked. (database is locked)
  HIL Write : quarc_library/Data Acquisition/Generic/Immediate I//O/HIL Write  object_name=HIL-1  analog_channels=[]  pwm_channels=[0:3]  digital_channels=[5:7 9:23]  other_channels=[]  sample_time=-1  active=off  vector_input=on
      settings: SourceProductName=The database C:\Users\user\AppData\Roaming\MathWorks\MATLAB\R2017a\slblocks_master.db is locked, or a table in the database is locked. (database is locked)
  Mux : Mux  Inputs=5
  Mux1 : Mux  Inputs=2
  Percent to quarter : Gain  Gain=125e-6
  Product : Product
  Red - Low Voltage Green - Armed Blue - Disarmed : Subsystem
  Sensor Failure Monitoring : Subsystem
  Sensor Data [6] : Outport
  DAQ Log : Outport  Port=2
  Battery Level (V) : Outport  Port=3
  wires:
  Percent to quarter/1 -> Bias - Pulse Offset (%)/1
  Arm (0,1)/1 -> Product/2, Red - Low Voltage Green - Armed Blue - Disarmed/1(Arm (0,1))
  "Battery Level, Accelrometer and Gyroscope"/2 -> Accel (m/s/s) [3]/1, Gyro (rad/s) [3]/1
  Check Battery level/1(Low Battery) -> Red - Low Voltage Green - Armed Blue - Disarmed/2(Low Battery (0,1)), Mux/3
  Sensor Failure Monitoring/1(Sensor Failure) -> Mux/1
  Mux/1 -> DAQ Log/1
  Accel (m/s/s) [3]/1 -> Mux/5, Mux1/2
  Gyro (rad/s) [3]/1 -> Mux/4, Mux1/1
  "Battery Level, Accelrometer and Gyroscope"/1 -> Conversion/1
  Mux1/1 -> Sensor Failure Monitoring/1(Sensor Data [6]), Sensor Data [6]/1
  Motor Cmd (%) [4]/1 -> Product/1
  Conversion/1 -> Mux/2, Battery Level (V)/1, Check Battery level/1(Battery level)
  Bias - Pulse Offset (%)/1 -> HIL Write/1
  Red - Low Voltage Green - Armed Blue - Disarmed/1(LEDs (%) [18]) -> HIL Write/2
  Product/1 -> Percent to quarter/1

== system Commander_Stabilizer_Qdrone_serial/STABILIZER - QDRONE /PIV CASCADE CONTROLLER1/MRFT_NEW  ==
  Error : Inport
  Enable : EnablePort
  Clock1 : Clock
  Constant5 : Constant  Value=-0.73
  Constant6 : Constant  Value=0.1
  Constant7 : Constant  Value=0.1
  Constant9 : Constant  Value=20
  MATLAB Function : MATLAB Function  TreatAsAtomicUnit=on
  control output : Outport
  wires:
  Constant7/1 -> MATLAB Function/4(no_switch_delay_in_s)
  Clock1/1 -> MATLAB Function/6(sim_time)
  Constant5/1 -> MATLAB Function/2(beta)
  Error/1 -> MATLAB Function/1(err)
  Constant9/1 -> MATLAB Function/5(num_of_peak_conf_samples)
  Constant6/1 -> MATLAB Function/3(h)
  MATLAB Function/1(output) -> control output/1  "control output"

== system Commander_Stabilizer_Qdrone_serial/STABILIZER - QDRONE /PIV CASCADE CONTROLLER1/MRFT_NEW 1 ==
  Error : Inport
  Enable : EnablePort
  Clock1 : Clock
  Constant5 : Constant  Value=-0.73
  Constant6 : Constant  Value=0.1
  Constant7 : Constant  Value=0.1
  Constant9 : Constant  Value=20
  MATLAB Function : MATLAB Function  TreatAsAtomicUnit=on
  control output : Outport
  wires:
  MATLAB Function/1(output) -> control output/1  "control output"
  Constant6/1 -> MATLAB Function/3(h)
  Constant9/1 -> MATLAB Function/5(num_of_peak_conf_samples)
  Error/1 -> MATLAB Function/1(err)
  Constant5/1 -> MATLAB Function/2(beta)
  Clock1/1 -> MATLAB Function/6(sim_time)
  Constant7/1 -> MATLAB Function/4(no_switch_delay_in_s)

== system Commander_Stabilizer_Qdrone_serial/STABILIZER - QDRONE /PIV CASCADE CONTROLLER1/PID  ==
  Error : Inport
  Roll rate : Inport  Port=2
  "reset " : Inport  Port=3
  Add : Sum  Inputs=++-
  Integrator1 : Integrator  ExternalReset=level  LimitOutput=on  UpperSaturationLimit=15*0.75  LowerSaturationLimit=-15*0.75
  Logical Operator : Logic  Operator=OR  AllPortsSameDT=off  OutDataTypeStr=boolean
  Logical Operator3 : Logic  Operator=NOT  AllPortsSameDT=off  OutDataTypeStr=boolean
  MATLAB Function1 : MATLAB Function  TreatAsAtomicUnit=on
  Product : Product
  Product1 : Product
  Product2 : Product
  Out1 : Outport
  wires:
  Error/1 -> Integrator1/1, Product/1
  Integrator1/1 -> Product2/2
  MATLAB Function1/3(Kd) -> Product1/1
  Roll rate/1 -> Product1/2
  Add/1 -> Out1/1
  Product1/1 -> Add/3
  MATLAB Function1/1(Kp) -> Product/2
  Product2/1 -> Add/2
  MATLAB Function1/2(Ki) -> Product2/1
  Product/1 -> Add/1
  [takeoff_cmd] -> Logical Operator3/1
  Logical Operator3/1 -> Logical Operator/2
  [roll_MRFT_MODE] -> Logical Operator/1
  Logical Operator/1 -> Integrator1/2

== system Commander_Stabilizer_Qdrone_serial/STABILIZER - QDRONE /PIV CASCADE CONTROLLER1/PID 1 ==
  Error : Inport
  Roll rate : Inport  Port=2
  "reset " : Inport  Port=3
  Add : Sum  Inputs=++-
  Integrator1 : Integrator  ExternalReset=level  LimitOutput=on  UpperSaturationLimit=15*0.75  LowerSaturationLimit=-15*0.75
  Logical Operator : Logic  Operator=OR  AllPortsSameDT=off  OutDataTypeStr=boolean
  Logical Operator3 : Logic  Operator=NOT  AllPortsSameDT=off  OutDataTypeStr=boolean
  MATLAB Function1 : MATLAB Function  TreatAsAtomicUnit=on
  Product : Product
  Product1 : Product
  Product2 : Product
  Out1 : Outport
  wires:
  Error/1 -> Integrator1/1, Product/1
  Integrator1/1 -> Product2/2
  MATLAB Function1/3(Kd) -> Product1/1
  Roll rate/1 -> Product1/2
  Add/1 -> Out1/1
  Product1/1 -> Add/3
  MATLAB Function1/1(Kp) -> Product/2
  Product2/1 -> Add/2
  MATLAB Function1/2(Ki) -> Product2/1
  Product/1 -> Add/1
  [takeoff_cmd] -> Logical Operator3/1
  Logical Operator3/1 -> Logical Operator/2
  [roll_MRFT_MODE] -> Logical Operator/1
  Logical Operator/1 -> Integrator1/2

== system Commander_Stabilizer_Qdrone_serial/STABILIZER - QDRONE /PIV CASCADE CONTROLLER1/PID yaw ==
  Error : Inport
  Roll rate : Inport  Port=2
  "reset " : Inport  Port=3
  Add : Sum  Inputs=++-
  Integrator1 : Integrator  ExternalReset=level  LimitOutput=on  UpperSaturationLimit=15*0.75  LowerSaturationLimit=-15*0.75
  Logical Operator : Logic  Operator=OR  AllPortsSameDT=off  OutDataTypeStr=boolean
  Logical Operator3 : Logic  Operator=NOT  AllPortsSameDT=off  OutDataTypeStr=boolean
  MATLAB Function1 : MATLAB Function  TreatAsAtomicUnit=on
  Product : Product
  Product1 : Product
  Product2 : Product
  Out1 : Outport
  wires:
  Error/1 -> Integrator1/1, Product/1
  Integrator1/1 -> Product2/2
  MATLAB Function1/3(Kd) -> Product1/1
  Roll rate/1 -> Product1/2
  Add/1 -> Out1/1
  Product1/1 -> Add/3
  MATLAB Function1/1(Kp) -> Product/2
  Product2/1 -> Add/2
  MATLAB Function1/2(Ki) -> Product2/1
  Product/1 -> Add/1
  [takeoff_cmd] -> Logical Operator3/1
  Logical Operator3/1 -> Logical Operator/2
  [roll_MRFT_MODE] -> Logical Operator/1
  Logical Operator/1 -> Integrator1/2
